simulink model "icttest"  (R2020b)
settings: Solver=VariableStepAuto  StartTime=0.0  StopTime=1  RelTol=1e-3
undefined symbols (not defined in the file or in its folder): f, spacar_lib, SPASIM
libraries: instrumentlib x2
settings Model: Creator=Rick  LastModifiedBy=Rick

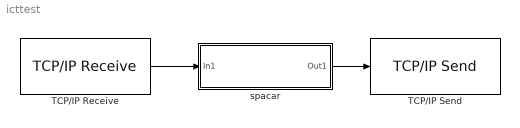
== system icttest ==
  TCP/IP Receive : instrumentlib/TCP//IP Receive  Host=127.0.0.1  Port=port  DataSize="[3  1]"  EnableBlockingMode=on  Timeout=10  SampleTime=0.01  DataType=double  ByteOrder=BigEndian  ASCIIFormatting=%f,  Terminator=LF
  TCP/IP Send : instrumentlib/TCP//IP Send  Host=127.0.0.1  Port=port  EnableBlockingMode=on  Timeout=10  ByteOrder=BigEndian  TransferDelay=on
  spacar : Subsystem  AncestorBlock=spacar_lib/SPASIM  mask{filename='bicycle', use_spadraw=off, output_sbd=off}
      mask prompts: filename "SPACAR data filename"; use_spadraw "Visualize with spadraw"; output_sbd "Write SBD file"
      mask init:
      | if size(who('filenm'))>0; dfilenm=filenm; else; dfilenm=''; end
      mask Display: disp(filename);
  wires:
  TCP/IP Receive/1 -> spacar/1(In1)
  spacar/1(Out1) -> TCP/IP Send/1

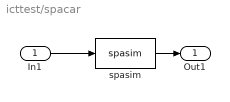
== system icttest/spacar ==
  In1 : Inport  PortDimensions=3
  spasim : S-Function  FunctionName=spasim  Parameters=filename,use_spadraw,output_sbd  SFunctionDeploymentMode=off  EnableBusSupport=off
  Out1 : Outport  InitialOutput=0  VectorParamsAs1DForOutWhenUnconnected=off
  wires:
  spasim/1 -> Out1/1
  In1/1 -> spasim/1
